simulink model "EMG_FES2_simulations"  (R2014a)
settings: Solver=FixedStepDiscrete  StartTime=0.0  StopTime=35  FixedStep=1/Fs  RelTol=1e-3
InitFcn:
  | load C:\SMSR1\activeFES-Feasibility\data\ap13\s1\best_calib\data_vars_clean.mat;
  | Fs=1000;%Hz
  | t=(1:length(EDC_emg))/Fs;
  | inputEMG=[t',EDC_emg,FDS_emg];
libraries: dspmtrx3 x8, dspinverses x4
settings Model: Creator=bethel.osuagwu  LastModifiedBy=bethel.osuagwu

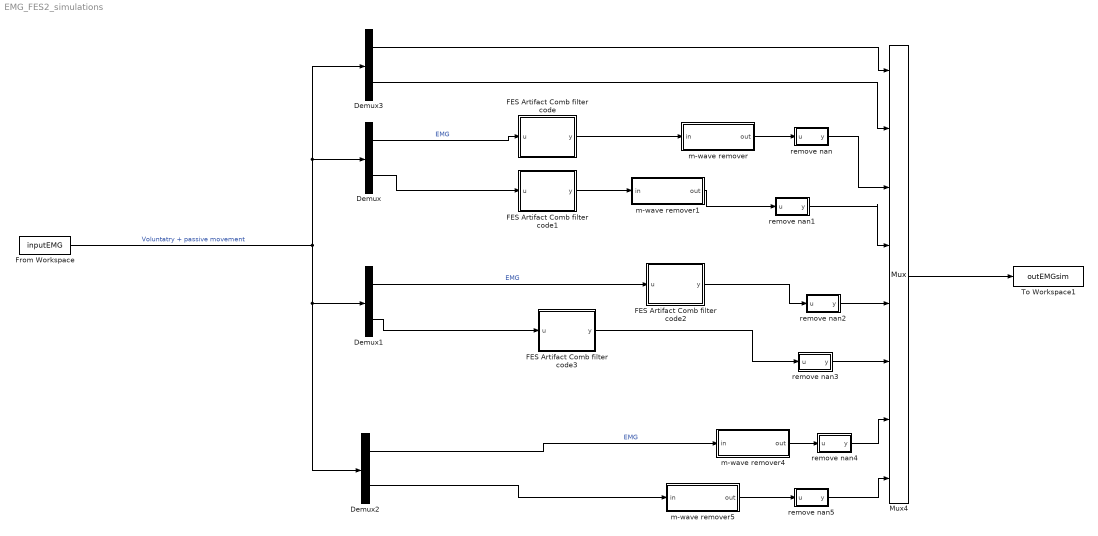
== system EMG_FES2_simulations ==
  Demux{,1..3} (4 alike) : Demux  Outputs=2
  FES Artifact Comb filter code : MATLAB Function  TreatAsAtomicUnit=on
  FES Artifact Comb filter code1 : MATLAB Function  TreatAsAtomicUnit=on
  FES Artifact Comb filter code2 : MATLAB Function  TreatAsAtomicUnit=on
  FES Artifact Comb filter code3 : MATLAB Function  TreatAsAtomicUnit=on
  From Workspace : FromWorkspace  VariableName=inputEMG  SampleTime=1/Fs  OutputAfterFinalValue=Setting to zero
  Mux4 : Mux  Inputs=8
  To Workspace1 : ToWorkspace  VariableName=outEMGsim  SampleTime=-1
  m-wave remover : Subsystem
  m-wave remover1 : Subsystem
  m-wave remover4 : Subsystem
  m-wave remover5 : Subsystem
  remove nan : MATLAB Function  TreatAsAtomicUnit=on
  remove nan1 : MATLAB Function  TreatAsAtomicUnit=on
  remove nan2 : MATLAB Function  TreatAsAtomicUnit=on
  remove nan3 : MATLAB Function  TreatAsAtomicUnit=on
  remove nan4 : MATLAB Function  TreatAsAtomicUnit=on
  remove nan5 : MATLAB Function  TreatAsAtomicUnit=on
  wires:
  Mux4/1 -> To Workspace1/1
  m-wave remover4/1(out) -> remove nan4/1(u)
  FES Artifact Comb filter code2/1(y) -> remove nan2/1(u)
  m-wave remover/1(out) -> remove nan/1(u)
  Demux3/2 -> Mux4/2
  Demux3/1 -> Mux4/1
  m-wave remover5/1(out) -> remove nan5/1(u)
  Demux2/2 -> m-wave remover5/1(in)
  Demux2/1 -> m-wave remover4/1(in)  "EMG"
  FES Artifact Comb filter code3/1(y) -> remove nan3/1(u)
  Demux1/2 -> FES Artifact Comb filter code3/1(u)
  Demux1/1 -> FES Artifact Comb filter code2/1(u)  "EMG"
  m-wave remover1/1(out) -> remove nan1/1(u)
  FES Artifact Comb filter code1/1(y) -> m-wave remover1/1(in)
  FES Artifact Comb filter code/1(y) -> m-wave remover/1(in)
  Demux/2 -> FES Artifact Comb filter code1/1(u)
  Demux/1 -> FES Artifact Comb filter code/1(u)  "EMG"
  remove nan/1(y) -> Mux4/3
  remove nan1/1(y) -> Mux4/4
  remove nan2/1(y) -> Mux4/5
  remove nan3/1(y) -> Mux4/6
  remove nan4/1(y) -> Mux4/7
  remove nan5/1(y) -> Mux4/8
  From Workspace/1 -> Demux1/1, Demux2/1, Demux3/1, Demux/1  "Voluntatry + passive movement"

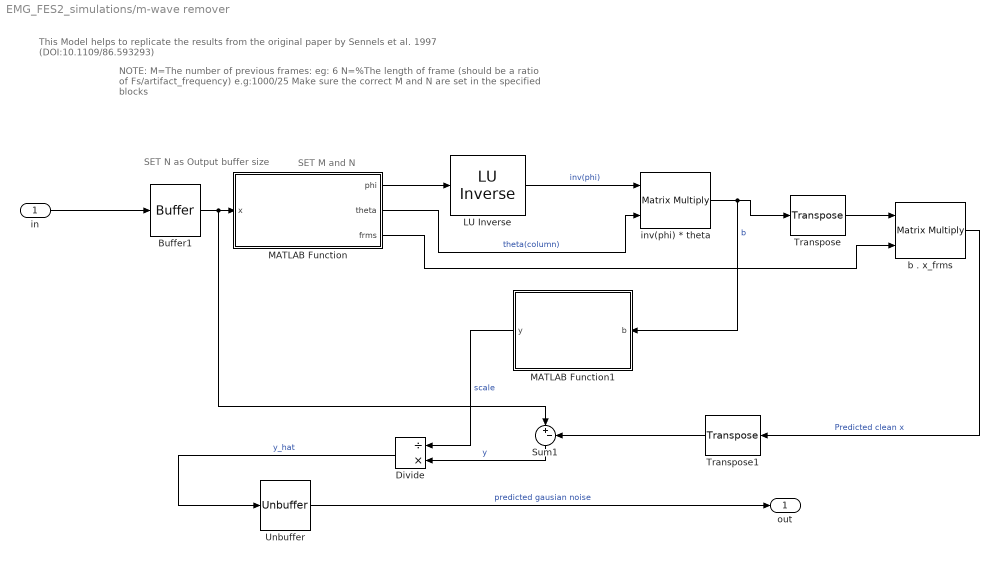
== system EMG_FES2_simulations/m-wave remover ==
  note: This Model helps to replicate the results from the original paper by Sennels et al. 1997 (DOI:10.1109/86.593293)
  note: SET M and N
  note: SET N as Output
      | buffer size
  note: NOTE:
      | M=The number of previous frames: eg: 6
      | N=%The length of frame (should be a ratio of Fs/artifact_frequency) e.g:1000/25
      | Make sure the correct M and N are set in the specified blocks
  in : Inport
  " LU Inverse" : dspinverses/ LU Inverse
  Buffer1 : Buffer  N=40  TreatMby1Signals=One channel
  Divide : Product  Inputs=/*
  MATLAB Function : MATLAB Function  TreatAsAtomicUnit=on
  MATLAB Function1 : MATLAB Function  TreatAsAtomicUnit=on
  Sum1 : Sum  Inputs=|+-
  Transpose : dspmtrx3/Transpose  Hermitian=off  overflowFlag=off
  Transpose1 : dspmtrx3/Transpose  Hermitian=off  overflowFlag=off
  Unbuffer : Unbuffer  SampleBasedProcessing=Same as frame based
  b . x_frms : Product  Multiplication=Matrix(*)
  inv(phi) * theta : Product  Multiplication=Matrix(*)
  out : Outport
  wires:
  in/1 -> Buffer1/1
  Divide/1 -> Unbuffer/1  "y_hat"
  MATLAB Function1/1(y) -> Divide/1  "scale"
  Sum1/1 -> Divide/2  "y"
  Transpose1/1 -> Sum1/2
  b . x_frms/1 -> Transpose1/1  "Predicted clean x"
  Transpose/1 -> b . x_frms/1
  MATLAB Function/3(frms) -> b . x_frms/2
  Unbuffer/1 -> out/1  "predicted gausian noise"
  inv(phi) * theta/1 -> Transpose/1, MATLAB Function1/1(b)  "b"
  " LU Inverse"/1 -> inv(phi) * theta/1  "inv(phi)"
  MATLAB Function/2(theta) -> inv(phi) * theta/2  "theta(column)"
  MATLAB Function/1(phi) -> " LU Inverse"/1
  Buffer1/1 -> MATLAB Function/1(x), Sum1/1

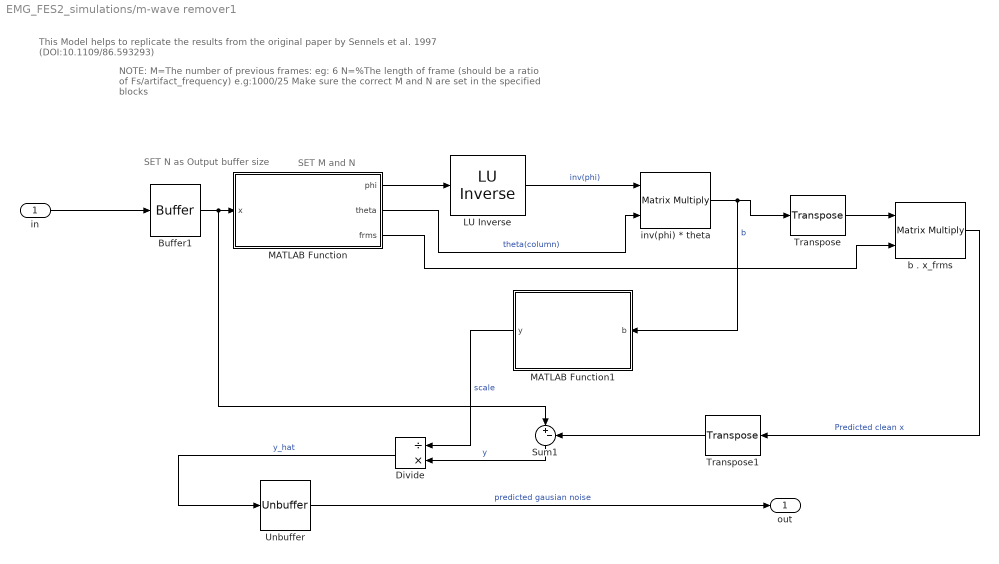
== system EMG_FES2_simulations/m-wave remover1 ==
  note: This Model helps to replicate the results from the original paper by Sennels et al. 1997 (DOI:10.1109/86.593293)
  note: SET M and N
  note: SET N as Output
      | buffer size
  note: NOTE:
      | M=The number of previous frames: eg: 6
      | N=%The length of frame (should be a ratio of Fs/artifact_frequency) e.g:1000/25
      | Make sure the correct M and N are set in the specified blocks
  in : Inport
  " LU Inverse" : dspinverses/ LU Inverse
  Buffer1 : Buffer  N=80  TreatMby1Signals=One channel
  Divide : Product  Inputs=/*
  MATLAB Function : MATLAB Function  TreatAsAtomicUnit=on
  MATLAB Function1 : MATLAB Function  TreatAsAtomicUnit=on
  Sum1 : Sum  Inputs=|+-
  Transpose : dspmtrx3/Transpose  Hermitian=off  overflowFlag=off
  Transpose1 : dspmtrx3/Transpose  Hermitian=off  overflowFlag=off
  Unbuffer : Unbuffer  SampleBasedProcessing=Same as frame based
  b . x_frms : Product  Multiplication=Matrix(*)
  inv(phi) * theta : Product  Multiplication=Matrix(*)
  out : Outport
  wires:
  in/1 -> Buffer1/1
  Divide/1 -> Unbuffer/1  "y_hat"
  MATLAB Function1/1(y) -> Divide/1  "scale"
  Sum1/1 -> Divide/2  "y"
  Transpose1/1 -> Sum1/2
  b . x_frms/1 -> Transpose1/1  "Predicted clean x"
  Transpose/1 -> b . x_frms/1
  MATLAB Function/3(frms) -> b . x_frms/2
  Unbuffer/1 -> out/1  "predicted gausian noise"
  inv(phi) * theta/1 -> Transpose/1, MATLAB Function1/1(b)  "b"
  " LU Inverse"/1 -> inv(phi) * theta/1  "inv(phi)"
  MATLAB Function/2(theta) -> inv(phi) * theta/2  "theta(column)"
  MATLAB Function/1(phi) -> " LU Inverse"/1
  Buffer1/1 -> MATLAB Function/1(x), Sum1/1

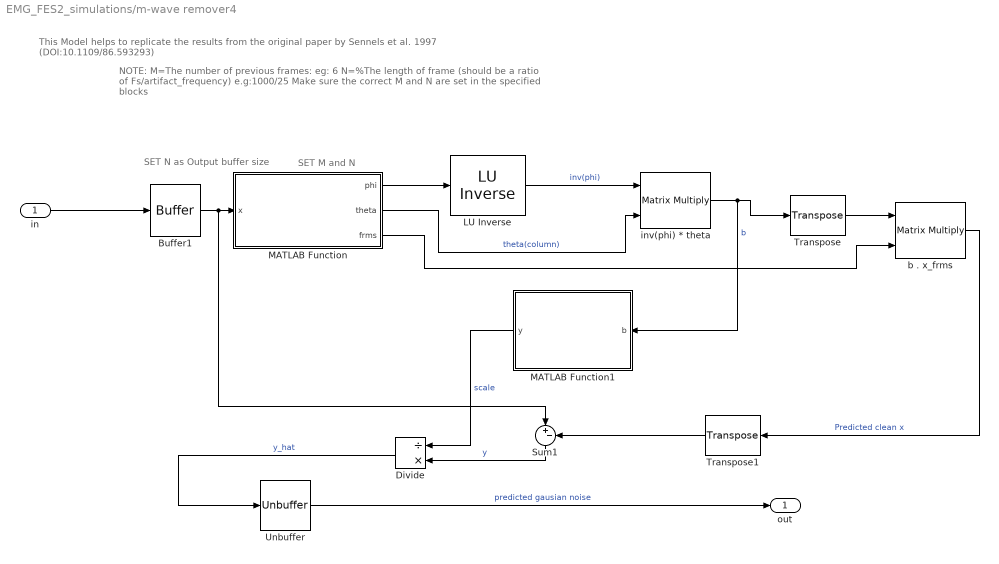
== system EMG_FES2_simulations/m-wave remover4 ==
  note: This Model helps to replicate the results from the original paper by Sennels et al. 1997 (DOI:10.1109/86.593293)
  note: SET M and N
  note: SET N as Output
      | buffer size
  note: NOTE:
      | M=The number of previous frames: eg: 6
      | N=%The length of frame (should be a ratio of Fs/artifact_frequency) e.g:1000/25
      | Make sure the correct M and N are set in the specified blocks
  in : Inport
  " LU Inverse" : dspinverses/ LU Inverse
  Buffer1 : Buffer  N=40  TreatMby1Signals=One channel
  Divide : Product  Inputs=/*
  MATLAB Function : MATLAB Function  TreatAsAtomicUnit=on
  MATLAB Function1 : MATLAB Function  TreatAsAtomicUnit=on
  Sum1 : Sum  Inputs=|+-
  Transpose : dspmtrx3/Transpose  Hermitian=off  overflowFlag=off
  Transpose1 : dspmtrx3/Transpose  Hermitian=off  overflowFlag=off
  Unbuffer : Unbuffer  SampleBasedProcessing=Same as frame based
  b . x_frms : Product  Multiplication=Matrix(*)
  inv(phi) * theta : Product  Multiplication=Matrix(*)
  out : Outport
  wires:
  in/1 -> Buffer1/1
  Divide/1 -> Unbuffer/1  "y_hat"
  MATLAB Function1/1(y) -> Divide/1  "scale"
  Sum1/1 -> Divide/2  "y"
  Transpose1/1 -> Sum1/2
  b . x_frms/1 -> Transpose1/1  "Predicted clean x"
  Transpose/1 -> b . x_frms/1
  MATLAB Function/3(frms) -> b . x_frms/2
  Unbuffer/1 -> out/1  "predicted gausian noise"
  inv(phi) * theta/1 -> Transpose/1, MATLAB Function1/1(b)  "b"
  " LU Inverse"/1 -> inv(phi) * theta/1  "inv(phi)"
  MATLAB Function/2(theta) -> inv(phi) * theta/2  "theta(column)"
  MATLAB Function/1(phi) -> " LU Inverse"/1
  Buffer1/1 -> MATLAB Function/1(x), Sum1/1

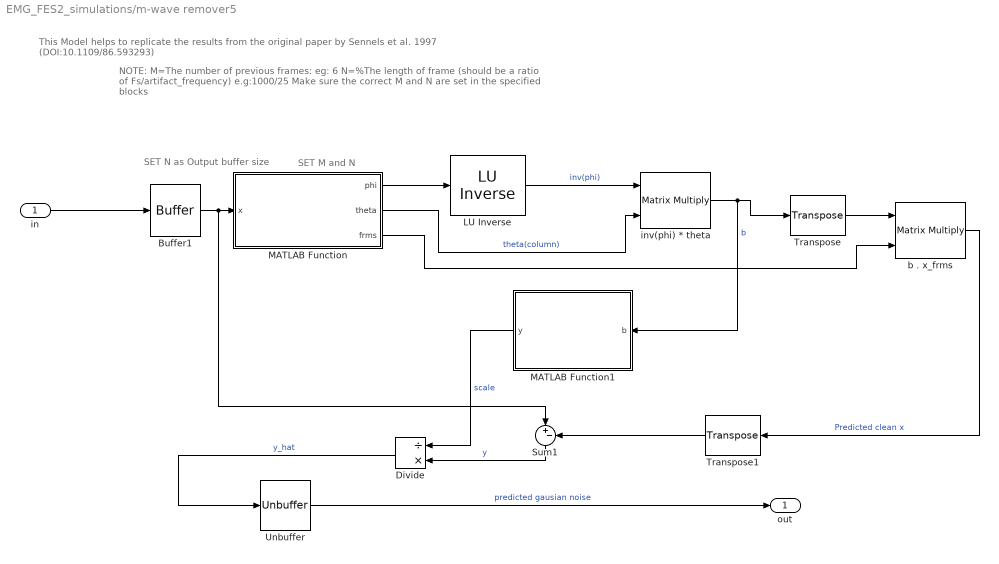
== system EMG_FES2_simulations/m-wave remover5 ==
  note: This Model helps to replicate the results from the original paper by Sennels et al. 1997 (DOI:10.1109/86.593293)
  note: SET M and N
  note: SET N as Output
      | buffer size
  note: NOTE:
      | M=The number of previous frames: eg: 6
      | N=%The length of frame (should be a ratio of Fs/artifact_frequency) e.g:1000/25
      | Make sure the correct M and N are set in the specified blocks
  in : Inport
  " LU Inverse" : dspinverses/ LU Inverse
  Buffer1 : Buffer  N=80  TreatMby1Signals=One channel
  Divide : Product  Inputs=/*
  MATLAB Function : MATLAB Function  TreatAsAtomicUnit=on
  MATLAB Function1 : MATLAB Function  TreatAsAtomicUnit=on
  Sum1 : Sum  Inputs=|+-
  Transpose : dspmtrx3/Transpose  Hermitian=off  overflowFlag=off
  Transpose1 : dspmtrx3/Transpose  Hermitian=off  overflowFlag=off
  Unbuffer : Unbuffer  SampleBasedProcessing=Same as frame based
  b . x_frms : Product  Multiplication=Matrix(*)
  inv(phi) * theta : Product  Multiplication=Matrix(*)
  out : Outport
  wires:
  in/1 -> Buffer1/1
  Divide/1 -> Unbuffer/1  "y_hat"
  MATLAB Function1/1(y) -> Divide/1  "scale"
  Sum1/1 -> Divide/2  "y"
  Transpose1/1 -> Sum1/2
  b . x_frms/1 -> Transpose1/1  "Predicted clean x"
  Transpose/1 -> b . x_frms/1
  MATLAB Function/3(frms) -> b . x_frms/2
  Unbuffer/1 -> out/1  "predicted gausian noise"
  inv(phi) * theta/1 -> Transpose/1, MATLAB Function1/1(b)  "b"
  " LU Inverse"/1 -> inv(phi) * theta/1  "inv(phi)"
  MATLAB Function/2(theta) -> inv(phi) * theta/2  "theta(column)"
  MATLAB Function/1(phi) -> " LU Inverse"/1
  Buffer1/1 -> MATLAB Function/1(x), Sum1/1

== matlab function EMG_FES2_simulations/FES Artifact Comb filter code ==
  data: u input; y output
function y  = fcn(u)
%#codegen

persistent u_mem;
fes_freq=25;%FES frequency
Fs=1000;%EMG/data samplerate
K=40;%round(Fs/fes_freq); %Comb filter order = (1/fes_freq)*Fs
a=-1;%{-1 to 0}
if isempty(u_mem)
    u_mem=zeros(K,1);
end





%% Comb filtering
% Forward comb
y=u+ a*u_mem(1);



u_mem(1:end-1)=u_mem(2:end);
u_mem(end)=u;



end





%

== matlab function EMG_FES2_simulations/remove nan1 ==
  data: u input; y output
function y  = fcn(u)
%#codegen

y=u;
if isnan(y)
    y=0;
end





%

== matlab function EMG_FES2_simulations/remove nan2 ==
  data: u input; y output
function y  = fcn(u)
%#codegen

y=u;
if isnan(y)
    y=0;
end





%

== matlab function EMG_FES2_simulations/remove nan3 ==
  data: u input; y output
function y  = fcn(u)
%#codegen

y=u;
if isnan(y)
    y=0;
end





%

== matlab function EMG_FES2_simulations/remove nan4 ==
  data: u input; y output
function y  = fcn(u)
%#codegen

y=u;
if isnan(y)
    y=0;
end





%

== matlab function EMG_FES2_simulations/remove nan5 ==
  data: u input; y output
function y  = fcn(u)
%#codegen

y=u;
if isnan(y)
    y=0;
end





%

== matlab function EMG_FES2_simulations/remove nan ==
  data: u input; y output
function y  = fcn(u)
%#codegen

y=u;
if isnan(y)
    y=0;
end





%

== matlab function EMG_FES2_simulations/FES Artifact Comb filter code1 ==
  data: u input; y output
function y  = fcn(u)
%#codegen

persistent u_mem;
fes_freq=25;%FES frequency
Fs=1000;%EMG/data samplerate
K=40;%round(Fs/fes_freq); %Comb filter order = (1/fes_freq)*Fs
a=-1;%{-1 to 0}
if isempty(u_mem)
    u_mem=zeros(K,1);
end





%% Comb filtering
% Forward comb
y=u+ a*u_mem(1);



u_mem(1:end-1)=u_mem(2:end);
u_mem(end)=u;
end





%

== matlab function EMG_FES2_simulations/FES Artifact Comb filter code2 ==
  data: u input; y output
function y  = fcn(u)
%#codegen

persistent u_mem;
fes_freq=25;%FES frequency
Fs=1000;%EMG/data samplerate
K=40;%round(Fs/fes_freq); %Comb filter order = (1/fes_freq)*Fs
a=-1;%{-1 to 0}
if isempty(u_mem)
    u_mem=zeros(K,1);
end





%% Comb filtering
% Forward comb
y=u+ a*u_mem(1);



u_mem(1:end-1)=u_mem(2:end);
u_mem(end)=u;



end





%

== matlab function EMG_FES2_simulations/FES Artifact Comb filter code3 ==
  data: u input; y output
function y  = fcn(u)
%#codegen

persistent u_mem;
fes_freq=25;%FES frequency
Fs=1000;%EMG/data samplerate
K=40;%round(Fs/fes_freq); %Comb filter order = (1/fes_freq)*Fs
a=-1;%{-1 to 0}
if isempty(u_mem)
    u_mem=zeros(K,1);
end





%% Comb filtering
% Forward comb
y=u+ a*u_mem(1);



u_mem(1:end-1)=u_mem(2:end);
u_mem(end)=u;
end





%

== matlab function EMG_FES2_simulations/m-wave remover/MATLAB Function ==
  data: x input; phi output double; theta output; frms output
function [phi,theta,frms] = fcn(x)
%#codegen
persistent t_sample phi_mem  frms_mem ;

%General param
M=6; %The number of previous frames 
N=40; %The length of frame (should be a ratio of Fs/artifact_frequency)

% Performance parameter
freshPhi =1;% when =1:recompute phi(covariance matix) all the phi; when =0:update phi with only new values

if isempty(t_sample)
    t_sample=0;
    frms_mem=zeros(M,N);
    
    phi_mem=zeros(M,M);
end
t_sample=t_sample+1;

%make x a row vector
x=x';


%% compute phi
frms=frms_mem;
%equ 7 and 8
if(freshPhi)
    % compute phi fresh all the time
    phi=(frms*frms');
else
    %we can compute only the required column (first) and row (first)of phi
    %matrix and push the new values into phi
    phi_mem(2:end,2:end)=phi_mem(1:end-1,1:end-1);
    phi_mem(1,:)=frms(1,:)*frms';
    phi_mem(:,1)=phi_mem(1,:)';
    %phi-phi_mem
    phi=phi_mem;
end


%% compute theta
theta=(x*frms')';
%t_sample
%if t_sample==15
%    y=4;
%end


%% update frame
frms_mem(2:end,:)=frms_mem(1:end-1,:);
frms_mem(1,:)=x;

== matlab function EMG_FES2_simulations/m-wave remover/MATLAB Function1 ==
  data: b input; y output
function y = fcn(b)
%#codegen


y = sqrt(1+sum(b.^2));
%       OR
%y = (1+sum(b));%approximated for speed

== matlab function EMG_FES2_simulations/m-wave remover1/MATLAB Function ==
  data: x input; phi output double; theta output; frms output
function [phi,theta,frms] = fcn(x)
%#codegen
persistent t_sample phi_mem  frms_mem ;

%General param
M=6; %The number of previous frames 
N=80; %The length of frame (should be a ratio of Fs/artifact_frequency)

% Performance parameter
freshPhi =1;% when =1:recompute phi(covariance matix) all the phi; when =0:update phi with only new values

if isempty(t_sample)
    t_sample=0;
    frms_mem=zeros(M,N);
    
    phi_mem=zeros(M,M);
end
t_sample=t_sample+1;

%make x a row vector
x=x';


%% compute phi
frms=frms_mem;
%equ 7 and 8
if(freshPhi)
    % compute phi fresh all the time
    phi=(frms*frms');
else
    %we can compute only the required column (first) and row (first)of phi
    %matrix and push the new values into phi
    phi_mem(2:end,2:end)=phi_mem(1:end-1,1:end-1);
    phi_mem(1,:)=frms(1,:)*frms';
    phi_mem(:,1)=phi_mem(1,:)';
    %phi-phi_mem
    phi=phi_mem;
end


%% compute theta
theta=(x*frms')';
%t_sample
%if t_sample==15
%    y=4;
%end


%% update frame
frms_mem(2:end,:)=frms_mem(1:end-1,:);
frms_mem(1,:)=x;

== matlab function EMG_FES2_simulations/m-wave remover1/MATLAB Function1 ==
  data: b input; y output
function y = fcn(b)
%#codegen


y = sqrt(1+sum(b.^2));
%       OR
%y = (1+sum(b));%approximated for speed

== matlab function EMG_FES2_simulations/m-wave remover4/MATLAB Function ==
  data: x input; phi output double; theta output; frms output
function [phi,theta,frms] = fcn(x)
%#codegen
persistent t_sample phi_mem  frms_mem ;

%General param
M=6; %The number of previous frames 
N=40; %The length of frame (should be a ratio of Fs/artifact_frequency)

% Performance parameter
freshPhi =1;% when =1:recompute phi(covariance matix) all the phi; when =0:update phi with only new values

if isempty(t_sample)
    t_sample=0;
    frms_mem=zeros(M,N);
    
    phi_mem=zeros(M,M);
end
t_sample=t_sample+1;

%make x a row vector
x=x';


%% compute phi
frms=frms_mem;
%equ 7 and 8
if(freshPhi)
    % compute phi fresh all the time
    phi=(frms*frms');
else
    %we can compute only the required column (first) and row (first)of phi
    %matrix and push the new values into phi
    phi_mem(2:end,2:end)=phi_mem(1:end-1,1:end-1);
    phi_mem(1,:)=frms(1,:)*frms';
    phi_mem(:,1)=phi_mem(1,:)';
    %phi-phi_mem
    phi=phi_mem;
end


%% compute theta
theta=(x*frms')';
%t_sample
%if t_sample==15
%    y=4;
%end


%% update frame
frms_mem(2:end,:)=frms_mem(1:end-1,:);
frms_mem(1,:)=x;

== matlab function EMG_FES2_simulations/m-wave remover4/MATLAB Function1 ==
  data: b input; y output
function y = fcn(b)
%#codegen


y = sqrt(1+sum(b.^2));
%       OR
%y = (1+sum(b));%approximated for speed

== matlab function EMG_FES2_simulations/m-wave remover5/MATLAB Function ==
  data: x input; phi output double; theta output; frms output
function [phi,theta,frms] = fcn(x)
%#codegen
persistent t_sample phi_mem  frms_mem ;

%General param
M=6; %The number of previous frames 
N=80; %The length of frame (should be a ratio of Fs/artifact_frequency)

% Performance parameter
freshPhi =1;% when =1:recompute phi(covariance matix) all the phi; when =0:update phi with only new values

if isempty(t_sample)
    t_sample=0;
    frms_mem=zeros(M,N);
    
    phi_mem=zeros(M,M);
end
t_sample=t_sample+1;

%make x a row vector
x=x';


%% compute phi
frms=frms_mem;
%equ 7 and 8
if(freshPhi)
    % compute phi fresh all the time
    phi=(frms*frms');
else
    %we can compute only the required column (first) and row (first)of phi
    %matrix and push the new values into phi
    phi_mem(2:end,2:end)=phi_mem(1:end-1,1:end-1);
    phi_mem(1,:)=frms(1,:)*frms';
    phi_mem(:,1)=phi_mem(1,:)';
    %phi-phi_mem
    phi=phi_mem;
end


%% compute theta
theta=(x*frms')';
%t_sample
%if t_sample==15
%    y=4;
%end


%% update frame
frms_mem(2:end,:)=frms_mem(1:end-1,:);
frms_mem(1,:)=x;

== matlab function EMG_FES2_simulations/m-wave remover5/MATLAB Function1 ==
  data: b input; y output
function y = fcn(b)
%#codegen


y = sqrt(1+sum(b.^2));
%       OR
%y = (1+sum(b));%approximated for speed
